simulink model "LookupTableDynamic3"  (R2014a)
settings: Solver=ode45  StartTime=0.0  StopTime=10.0  RelTol=1e-3
libraries: simulink x1
settings Model: CovSFcnEnable=on  BufferReuse=off  Creator=yamasefu  LastModifiedBy=ts1413
settings OptimizationCC: SimCompilerOptimization=off
settings DebuggingCC: MergeDetectMultiDrivingBlocksExec=error  SolverPrmCheckMsg=none  FrameProcessingCompatibilityMsg=error
settings RTWCC: RTWCompilerOptimization=off

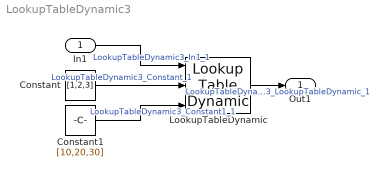
== system LookupTableDynamic3 ==
  In1 : Inport
  Constant : Constant  Value=[1,2,3]
  Constant1 : Constant  Value=[10,20,30]
  LookupTableDynamic : simulink/Lookup Tables/Lookup Table Dynamic  LookUpMeth=Use Input Nearest  OutDataTypeStr=fixdt('double')  OutputDataTypeScalingMode=Specify via dialog  OutDataType=fixdt('double')  OutScaling=2^-10  DoSatur=off
  Out1 : Outport
  wires:
  In1/1 -> LookupTableDynamic/1  "LookupTableDynamic3_In1_1"
  Constant/1 -> LookupTableDynamic/2  "LookupTableDynamic3_Constant_1"
  Constant1/1 -> LookupTableDynamic/3  "LookupTableDynamic3_Constant1_1"
  LookupTableDynamic/1 -> Out1/1  "LookupTableDynamic3_LookupTableDynamic_1"
